simulink model "torque_allocator"  (R2023a)
settings: Solver=VariableStepAuto  StartTime=0.0  StopTime=20  RelTol=1e-3
settings Model: Creator=pablo  LastModifiedBy=pablo

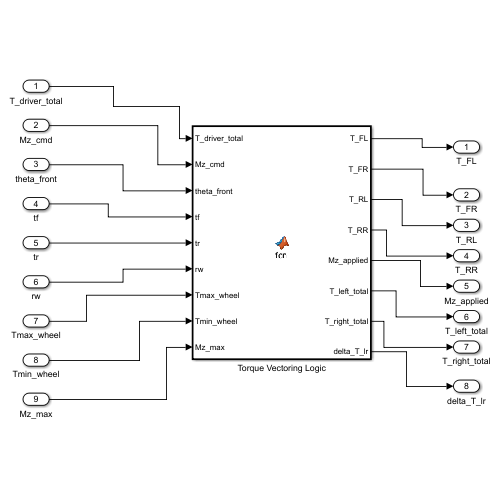
[thumbnail: Simulink's stored preview of the top-level diagram]
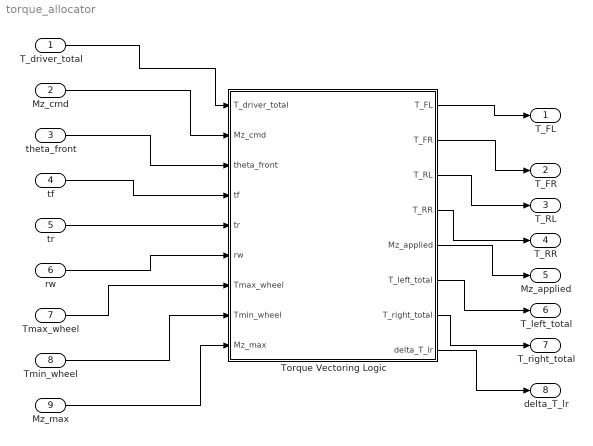
== system torque_allocator ==
  T_driver_total : Inport
  Mz_cmd : Inport  Port=2
  theta_front : Inport  Port=3
  tf : Inport  Port=4
  tr : Inport  Port=5
  rw : Inport  Port=6
  Tmax_wheel : Inport  Port=7
  Tmin_wheel : Inport  Port=8
  Mz_max : Inport  Port=9
  Torque Vectoring Logic : MATLAB Function  TreatAsAtomicUnit=on
  T_FL : Outport
  T_FR : Outport  Port=2
  T_RL : Outport  Port=3
  T_RR : Outport  Port=4
  Mz_applied : Outport  Port=5
  T_left_total : Outport  Port=6
  T_right_total : Outport  Port=7
  delta_T_lr : Outport  Port=8
  wires:
  T_driver_total/1 -> Torque Vectoring Logic/1(T_driver_total)
  Mz_cmd/1 -> Torque Vectoring Logic/2(Mz_cmd)
  theta_front/1 -> Torque Vectoring Logic/3(theta_front)
  tf/1 -> Torque Vectoring Logic/4(tf)
  tr/1 -> Torque Vectoring Logic/5(tr)
  rw/1 -> Torque Vectoring Logic/6(rw)
  Tmax_wheel/1 -> Torque Vectoring Logic/7(Tmax_wheel)
  Tmin_wheel/1 -> Torque Vectoring Logic/8(Tmin_wheel)
  Mz_max/1 -> Torque Vectoring Logic/9(Mz_max)
  Torque Vectoring Logic/1(T_FL) -> T_FL/1
  Torque Vectoring Logic/2(T_FR) -> T_FR/1
  Torque Vectoring Logic/3(T_RL) -> T_RL/1
  Torque Vectoring Logic/4(T_RR) -> T_RR/1
  Torque Vectoring Logic/5(Mz_applied) -> Mz_applied/1
  Torque Vectoring Logic/6(T_left_total) -> T_left_total/1
  Torque Vectoring Logic/7(T_right_total) -> T_right_total/1
  Torque Vectoring Logic/8(delta_T_lr) -> delta_T_lr/1

== matlab function torque_allocator/Torque Vectoring Logic ==
  data: T_driver_total input; T_FL output; Mz_cmd input; theta_front input; tf input; tr input; rw input; Tmax_wheel input; Tmin_wheel input; Mz_max input; T_FR output; T_RL output; T_RR output; Mz_applied output; T_left_total output; T_right_total output; delta_T_lr output
function [T_FL, T_FR, T_RL, T_RR, Mz_applied, T_left_total, T_right_total, delta_T_lr] = fcn(T_driver_total, Mz_cmd, theta_front, tf, tr, rw, Tmax_wheel, Tmin_wheel, Mz_max)

% Saturate requested yaw moment
if Mz_cmd > Mz_max
    Mz_cmd = Mz_max;
elseif Mz_cmd < -Mz_max
    Mz_cmd = -Mz_max;
end

% Nominal symmetric torque distribution
T_nom = T_driver_total / 4;

T_FL_nom = T_nom;
T_FR_nom = T_nom;
T_RL_nom = T_nom;
T_RR_nom = T_nom;

% Split yaw moment between front and rear axle
Mz_front = theta_front * Mz_cmd;
Mz_rear  = (1 - theta_front) * Mz_cmd;

% Convert yaw moment into left-right torque difference
dT_front = (Mz_front * rw) / tf;
dT_rear  = (Mz_rear  * rw) / tr;

% Positive Mz: more torque on right wheels, less on left wheels
T_FL = T_FL_nom - dT_front;
T_FR = T_FR_nom + dT_front;
T_RL = T_RL_nom - dT_rear;
T_RR = T_RR_nom + dT_rear;

% Wheel torque saturation
T_FL = min(max(T_FL, Tmin_wheel), Tmax_wheel);
T_FR = min(max(T_FR, Tmin_wheel), Tmax_wheel);
T_RL = min(max(T_RL, Tmin_wheel), Tmax_wheel);
T_RR = min(max(T_RR, Tmin_wheel), Tmax_wheel);

% Estimate actually generated yaw moment after saturation
Fx_FL = T_FL / rw;
Fx_FR = T_FR / rw;
Fx_RL = T_RL / rw;
Fx_RR = T_RR / rw;

Mz_front_applied = (Fx_FR - Fx_FL) * tf / 2;
Mz_rear_applied  = (Fx_RR - Fx_RL) * tr / 2;

Mz_applied = Mz_front_applied + Mz_rear_applied;

% Additional outputs for analysis and plots
T_left_total  = T_FL + T_RL;
T_right_total = T_FR + T_RR;
delta_T_lr    = T_right_total - T_left_total;

end
